simulink model "Linear_model"  (R2024a)
settings: Solver=VariableStepAuto  StartTime=0.0  StopTime=10.0  RelTol=1e-3
values from neighbouring files (symbols this model uses):
  A = [-(Cyf + Cyr)/(m*Vx0) (-lf*Cyf + lr*Cyr)/(m*Vx0) - Vx0 ... (first row only)    [model_param.m]
  B = [Cyf/(m*V   x0) 0 ... (first row only)    [model_param.m]
  C = eye(2)    [model_param.m]
  D = zeros(2,2)    [model_param.m]
settings Model: Creator=dydtj  LastModifiedBy=dydtj

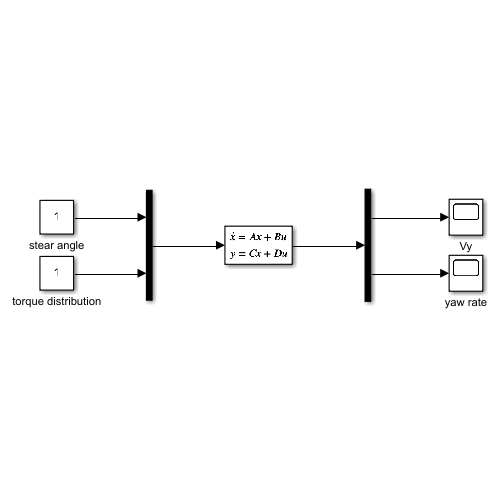
[thumbnail: Simulink's stored preview of the top-level diagram]
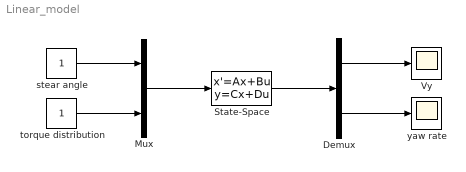
== system Linear_model ==
  Demux : Demux  Outputs=2
  Mux : Mux  Inputs=2
  State-Space : StateSpace  A=A  B=B  C=C  D=D  InitialCondition=0
  Vy : Scope
  stear angle : Constant
  torque distribution : Constant
  yaw rate : Scope
  wires:
  Mux/1 -> State-Space/1
  stear angle/1 -> Mux/1
  torque distribution/1 -> Mux/2
  State-Space/1 -> Demux/1
  Demux/1 -> Vy/1
  Demux/2 -> yaw rate/1
